simulink model "Model0"  (R2023b)
settings: Solver=VariableStepAuto  StartTime=0.0  StopTime=10.0  RelTol=1e-3
values from neighbouring files (symbols this model uses):
  A = pi*((d)^2)/4    (= 0.196349540849)    [Parameters.m]
  a = 2.2*10^-4    (= 0.00022)    [Parameters.m]
  Af = 45    [Parameters.m]
  As = 30    [Parameters.m]
  c = c_*A/L_SMA    (= 0.00981747704247)    [Parameters.m]
  c_ = 10    [Parameters.m]
  Ca = 10.3    [Parameters.m]
  Cm = 7    [Parameters.m]
  Cp = 322    [Parameters.m]
  d = 0.5    [Parameters.m]
  e_l = 0.05    [Parameters.m]
  Ea = 75000    [Parameters.m]
  Em = 28000    [Parameters.m]
  gm = I_max/V_max    (= 0.945945945946)    [Parameters.m]
  h = 36200    [Parameters.m]
  Ip = a*T0/Rp    (= 0.00210434782609)    [Parameters.m]
  k = k_*Ap/t    (= 4.26315789474)    [Parameters.m]
  L_SMA = 200    [Parameters.m]
  m = (V*10^-9)/raw    (= 6.08835785579e-12)    [Parameters.m]
  n = 3    [Parameters.m]
  R = 7.8    [Parameters.m]
  R1 = 1000    [Parameters.m]
  R2 = 1000    [Parameters.m]
  R_ = 0.000820    (= 0.00082)    [Parameters.m]
  R_load = Gv/gm    (= 2.11428571429)    [Parameters.m]
  Rp = 2.3    [Parameters.m]
  T0 = 22    [Parameters.m]
undefined symbols (not defined in the file or in its folder): K, R_int, T
libraries: fl_lib x4, ee_lib x2, nesl_utility x2
settings Model: Creator=DELL  LastModifiedBy=DELL

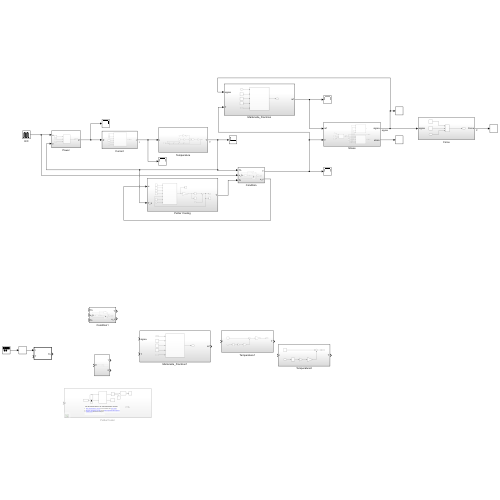
[thumbnail: Simulink's stored preview of the top-level diagram]
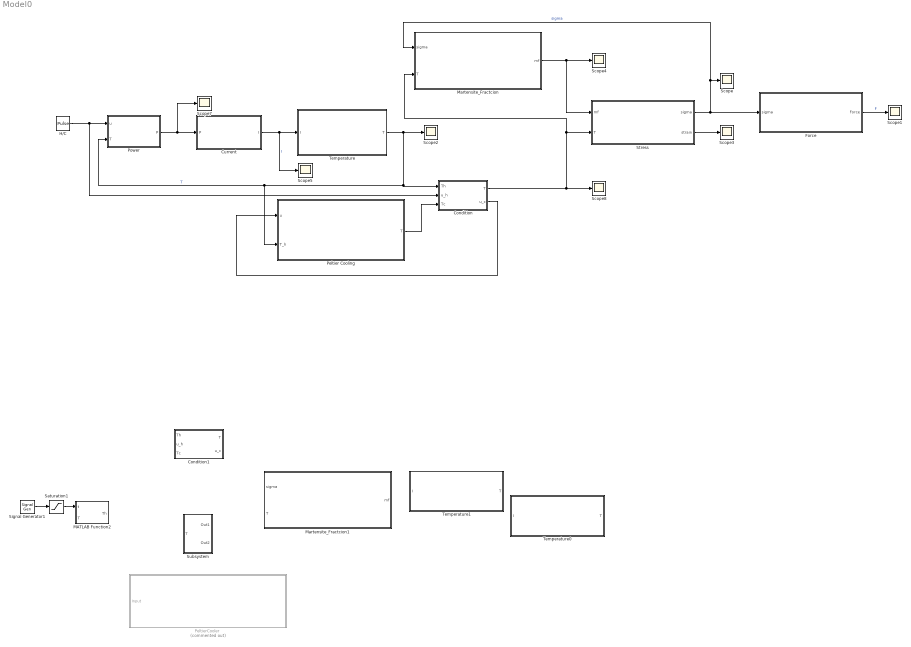
== system Model0 ==
  Condition : Subsystem
  Condition1 : Subsystem
  Current : Subsystem
  Force : Subsystem
  H/C : DiscretePulseGenerator  PulseType=Time based  Period=10  PulseWidth=50
  MATLAB Function2 : MATLAB Function  TreatAsAtomicUnit=on
  Martensite_Fractcion : Subsystem
  Martensite_Fractcion1 : Subsystem
  Peltier Cooling : Subsystem
  PeltierCooler : Subsystem  Commented=on
  Power : Subsystem
  Saturation1 : Saturate  UpperLimit=0.0578  LowerLimit=0
  Scope{,1..5,7..8} (8 alike) : Scope
  Signal Generator1 : SignalGenerator  WaveForm=square  Amplitude=-0.0578  Frequency=0.095
  Stress : Subsystem
  Subsystem : Subsystem
  Temperature : Subsystem
  Temperature0 : Subsystem
  Temperature1 : Subsystem
  wires:
  Martensite_Fractcion/1(mf) -> Scope4/1, Stress/1(mf)
  Stress/1(sigma) -> Martensite_Fractcion/1(sigma), Scope/1, Force/1(sigma)  "sigma"
  Force/1(Force) -> Scope1/1  "F"
  Temperature/1(T) -> Scope2/1, Peltier Cooling/2(T_h), Power/2(T), Condition/1(Th)  "T"
  Current/1(I) -> Temperature/1(I), Scope5/1  "I"
  Stress/2(strain) -> Scope3/1
  Signal Generator1/1 -> Saturation1/1
  Saturation1/1 -> MATLAB Function2/1(t)
  Condition/1(T) -> Martensite_Fractcion/2(T), Stress/2(T), Scope8/1
  Peltier Cooling/1(T) -> Condition/3(Tc)
  Condition/2(u_c) -> Peltier Cooling/1(u)
  Power/1(P) -> Scope7/1, Current/1(P)
  H/C/1 -> Condition/2(u_h), Power/1(u)

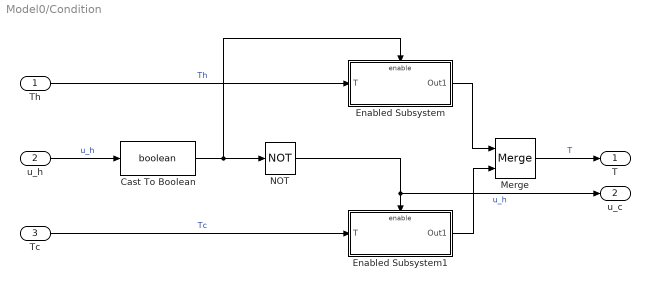
== system Model0/Condition ==
  Th : Inport
  u_h : Inport  Port=2
  Tc : Inport  Port=3
  Cast To Boolean : DataTypeConversion  OutDataTypeStr=boolean  SaturateOnIntegerOverflow=off  RndMeth=Floor
  Enabled Subsystem : Subsystem  TreatAsAtomicUnit=on
  Enabled Subsystem1 : Subsystem  TreatAsAtomicUnit=on
  Merge : Merge
  NOT : Logic  Operator=NOT  IconShape=distinctive  AllPortsSameDT=off  OutDataTypeStr=boolean
  T : Outport
  u_c : Outport  Port=2
  wires:
  Merge/1 -> T/1  "T"
  Enabled Subsystem/1(Out1) -> Merge/1
  Cast To Boolean/1 -> NOT/1, Enabled Subsystem/Enable
  NOT/1 -> u_c/1, Enabled Subsystem1/Enable  "u_h"
  Tc/1 -> Enabled Subsystem1/1(T)  "Tc"
  Th/1 -> Enabled Subsystem/1(T)  "Th"
  Enabled Subsystem1/1(Out1) -> Merge/2
  u_h/1 -> Cast To Boolean/1  "u_h"

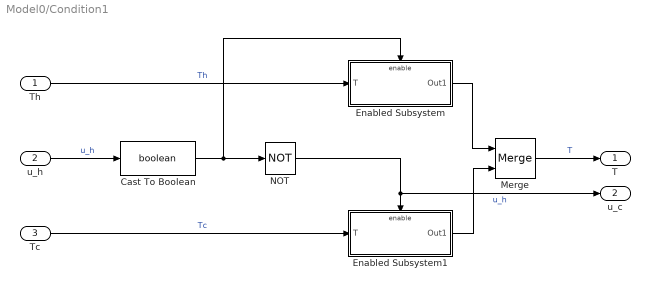
== system Model0/Condition1 ==
  Th : Inport
  u_h : Inport  Port=2
  Tc : Inport  Port=3
  Cast To Boolean : DataTypeConversion  OutDataTypeStr=boolean  SaturateOnIntegerOverflow=off  RndMeth=Floor
  Enabled Subsystem : Subsystem  TreatAsAtomicUnit=on
  Enabled Subsystem1 : Subsystem  TreatAsAtomicUnit=on
  Merge : Merge
  NOT : Logic  Operator=NOT  IconShape=distinctive  AllPortsSameDT=off  OutDataTypeStr=boolean
  T : Outport
  u_c : Outport  Port=2
  wires:
  Merge/1 -> T/1  "T"
  Enabled Subsystem/1(Out1) -> Merge/1
  Cast To Boolean/1 -> NOT/1, Enabled Subsystem/Enable
  NOT/1 -> u_c/1, Enabled Subsystem1/Enable  "u_h"
  Tc/1 -> Enabled Subsystem1/1(T)  "Tc"
  Th/1 -> Enabled Subsystem/1(T)  "Th"
  Enabled Subsystem1/1(Out1) -> Merge/2
  u_h/1 -> Cast To Boolean/1  "u_h"

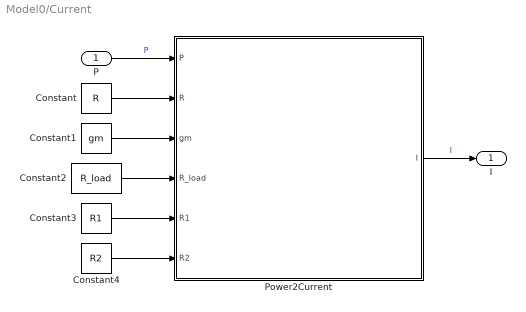
== system Model0/Current ==
  P : Inport
  Constant : Constant  Value=R
  Constant1 : Constant  Value=gm
  Constant2 : Constant  Value=R_load
  Constant3 : Constant  Value=R1
  Constant4 : Constant  Value=R2
  Power2Current : MATLAB Function  TreatAsAtomicUnit=on
  I : Outport
  wires:
  P/1 -> Power2Current/1(P)  "P"
  Power2Current/1(I) -> I/1  "I"
  Constant/1 -> Power2Current/2(R)
  Constant2/1 -> Power2Current/4(R_load)
  Constant3/1 -> Power2Current/5(R1)
  Constant4/1 -> Power2Current/6(R2)
  Constant1/1 -> Power2Current/3(gm)

== system Model0/Force ==
  sigma : Inport
  Area_SMA : Constant  Value=A
  Divide : Product  Inputs=***
  No. of Wires : Constant  Value=n
  Force : Outport
  wires:
  Area_SMA/1 -> Divide/2  "A"
  sigma/1 -> Divide/3  "sigma"
  Divide/1 -> Force/1  "F"
  No. of Wires/1 -> Divide/1  "n"

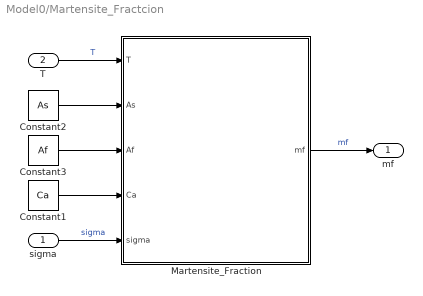
== system Model0/Martensite_Fractcion ==
  sigma : Inport
  T : Inport  Port=2
  Constant1 : Constant  Value=Ca
  Constant2 : Constant  Value=As
  Constant3 : Constant  Value=Af
  Martensite_Fraction : MATLAB Function  TreatAsAtomicUnit=on
  mf : Outport
  wires:
  sigma/1 -> Martensite_Fraction/5(sigma)  "sigma"
  Constant2/1 -> Martensite_Fraction/2(As)
  Martensite_Fraction/1(mf) -> mf/1  "mf"
  T/1 -> Martensite_Fraction/1(T)  "T"
  Constant1/1 -> Martensite_Fraction/4(Ca)
  Constant3/1 -> Martensite_Fraction/3(Af)

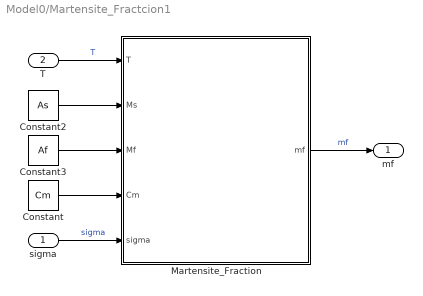
== system Model0/Martensite_Fractcion1 ==
  sigma : Inport
  T : Inport  Port=2
  Constant : Constant  Value=Cm
  Constant2 : Constant  Value=As
  Constant3 : Constant  Value=Af
  Martensite_Fraction : MATLAB Function  TreatAsAtomicUnit=on
  mf : Outport
  wires:
  sigma/1 -> Martensite_Fraction/5(sigma)  "sigma"
  Constant2/1 -> Martensite_Fraction/2(Ms)
  Martensite_Fraction/1(mf) -> mf/1  "mf"
  T/1 -> Martensite_Fraction/1(T)  "T"
  Constant/1 -> Martensite_Fraction/4(Cm)
  Constant3/1 -> Martensite_Fraction/3(Mf)

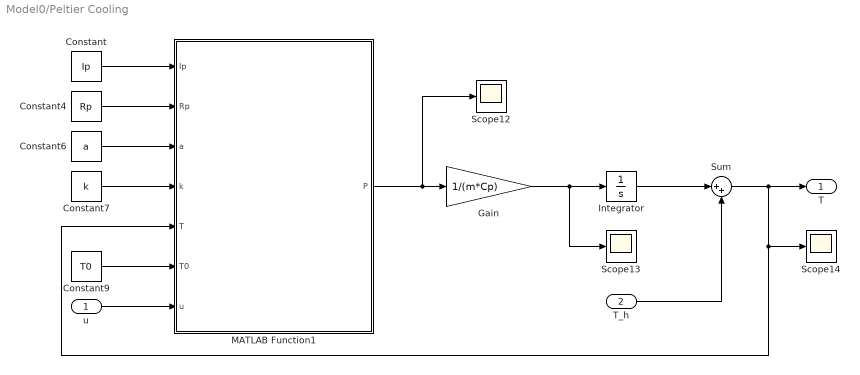
== system Model0/Peltier Cooling ==
  u : Inport
  T_h : Inport  Port=2
  Constant : Constant  Value=Ip
  Constant4 : Constant  Value=Rp
  Constant6 : Constant  Value=a
  Constant7 : Constant  Value=k
  Constant9 : Constant  Value=T0
  Gain : Gain  Gain=1/(m*Cp)
  Integrator : Integrator
  MATLAB Function1 : MATLAB Function  TreatAsAtomicUnit=on
  Scope12 : Scope
  Scope13 : Scope
  Scope14 : Scope
  Sum : Sum  Inputs=|++
  T : Outport
  wires:
  Constant4/1 -> MATLAB Function1/2(Rp)
  MATLAB Function1/1(P) -> Scope12/1, Gain/1
  Constant6/1 -> MATLAB Function1/3(a)
  T_h/1 -> Sum/2
  u/1 -> MATLAB Function1/7(u)
  Constant9/1 -> MATLAB Function1/6(T0)
  Constant/1 -> MATLAB Function1/1(Ip)
  Integrator/1 -> Sum/1
  Sum/1 -> T/1, MATLAB Function1/5(T), Scope14/1
  Gain/1 -> Scope13/1, Integrator/1
  Constant7/1 -> MATLAB Function1/4(k)

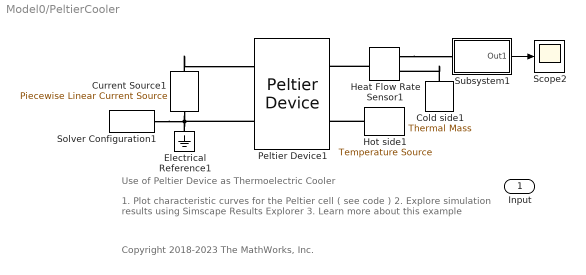
== system Model0/PeltierCooler ==
  note: Copyright 2018-2023 The MathWorks, Inc.
  note: 1. Plot characteristic curves for the Peltier cell ( see code )
      | 2. Explore simulation results using Simscape Results Explorer
      | 3. Learn more about this example
  note: Use of Peltier Device as Thermoelectric Cooler
  Input : Inport
  Cold side1 : fl_lib/Thermal/Thermal Elements/Thermal Mass  mass_type=foundation.enum.constant_variable.constant  mass=1 kg  sp_heat=447 J/kg/K  mass_min=1e-6 kg  num_ports=foundation.enum.numPorts2.one  m_specify=off  m_priority=High  m=1 kg  m_nominal_specify=off  m_nominal_unit=kg  m_nominal_value=1  T_specify=on  T_priority=High  T=T K  T_nominal_specify=off  T_nominal_unit=K  T_nominal_value=1  Q_specify=off  Q_priority=None  Q=0 W  Q_nominal_specify=off  Q_nominal_unit=W  Q_nominal_value=1
  Current Source1 : ee_lib/Additional Components/SPICE Sources/Piecewise Linear Current Source  TIMElist=[0, 10] s  CURRlist=[0.01, 5.5] A  INTERP=1  EXTRAP=1  Gmin_param=ee.enum.gminParam.yes
      settings: InternalSimscapePortConfiguration="{\"Bottom\":[],\"Left\":[{\"id\":\"p\",\"label\":\"+\",\"type\":\"foundation.electrical.electrical\"}],\"Right\":[{\"id\":\"n\",\"label\":\"-\",\"type\":\"foundation.electrical.electrical\"}],\"Top\":[]}"
  Electrical Reference1 : fl_lib/Electrical/Electrical Elements/Electrical Reference
  Heat Flow Rate Sensor1 : fl_lib/Thermal/Thermal Sensors/Heat Flow Rate Sensor
  Hot side1 : fl_lib/Thermal/Thermal Sources/Temperature Source  temperature=323.15 K
  Peltier Device1 : ee_lib/Sensors & Transducers/Peltier Device  alpha="coef  V/K"  R="R_int  Ohm"  K=K W/K
      settings: InternalSimscapePortConfiguration="{\"Bottom\":[],\"Left\":[{\"id\":\"p\",\"label\":\"+\",\"type\":\"foundation.electrical.electrical\"},{\"id\":\"n\",\"label\":\"-\",\"type\":\"foundation.electrical.electrical\"}],\"Right\":[{\"id\":\"A\",\"label\":\"A\",\"type\":\"foundation.thermal.thermal\"},{\"id\":\"B\",\"label\":\"B\",\"type\":\"foundation.thermal.thermal\"}],\"Top\":[]}"
  Scope2 : Scope
  Solver Configuration1 : nesl_utility/Solver Configuration  PhysicalDomain=network_engine_domain  SubClassName=solver  LeftPortType=input  RightPortType=generic  Tones=[]  Harmonics=[]  SimulateNoise=off  Profile=off  UseLocalSampling=off  EnableSwitchedLinearOptims=on  FrequencyDomain=off  UseCCode=off  RelTol=0.001  AbsTol=1e-06  MinStep=1e-09  ToWorkspace=off  RevertToSquareIcSolve=off  NumHomotopyIterations=100  PhasorMode=off  PhasorModeNumHarmonics=1  ConsistencySolver=NEWTON_FTOL  IndexReductionMethod=DerivativeReplacement  DoDC=off  ResidualTolerance=1e-09  ConsistencyTolSource=GLOBAL  ConsistencyAbsTol=0.001  ConsistencyRelTol=0.001  ConsistencyTolFactor=0.001  UseLocalSolver=off  LocalSolverChoice=NE_BACKWARD_EULER_ADVANCER  ResolveIndetEquations=on  FunctionEvalNumThread=1  LocalSolverSampleTime=0.001  DoFixedCost=off  MaxNonlinIter=3  MaxModeIter=2  ComputeImpulses=off  ImpulseIterations=2  LinearAlgebra=auto  LinearAlgebraNumThread=0  EquationFormulation=NE_TIME_EF  DelaysMemoryBudget=1024  AutomaticFiltering=on  FilteringTimeConstant=0.001  PartitionStorageMethod=AS_NEEDED  PartitionMemoryBudget=1024  PartitionMethod=FAST  MultibodyUseLocalSolver=off  MultibodyLocalSolverChoice=ODE1  MultibodyLocalSolverSampleTime=0.001
  Subsystem1 : Subsystem
      mask Display: disp('Heat flow')
  wires:
  Subsystem1/1(Out1) -> Scope2/1
  connections:
  Heat Flow Rate Sensor1/LConn1 -- Peltier Device1/RConn1
  Current Source1/LConn1 -- Solver Configuration1/RConn1 -- Electrical Reference1/LConn1 -- Peltier Device1/LConn2
  Heat Flow Rate Sensor1/RConn1 -- Subsystem1/LConn1
  Cold side1/LConn1 -- Heat Flow Rate Sensor1/RConn2
  Hot side1/LConn1 -- Peltier Device1/RConn2
  Current Source1/RConn1 -- Peltier Device1/LConn1

== system Model0/Power ==
  u : Inport
  T : Inport  Port=2
  MATLAB Function1 : MATLAB Function  TreatAsAtomicUnit=on
  Step : Step  After=0.0578  SampleTime=0
  P : Outport
  wires:
  T/1 -> MATLAB Function1/3(T)  "T"
  MATLAB Function1/1(P) -> P/1  "P"
  Step/1 -> MATLAB Function1/1(p)  "P"
  u/1 -> MATLAB Function1/2(u)  "u"

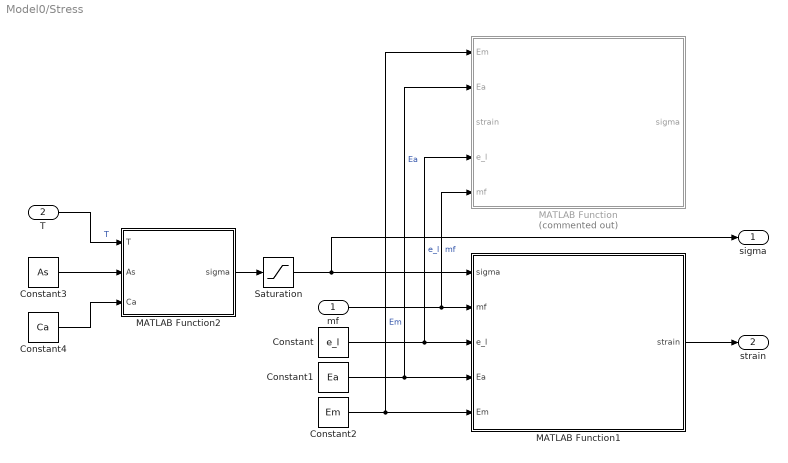
== system Model0/Stress ==
  mf : Inport
  T : Inport  Port=2
  Constant : Constant  Value=e_l
  Constant1 : Constant  Value=Ea
  Constant2 : Constant  Value=Em
  Constant3 : Constant  Value=As
  Constant4 : Constant  Value=Ca
  MATLAB Function : MATLAB Function  Commented=on  TreatAsAtomicUnit=on
  MATLAB Function1 : MATLAB Function  TreatAsAtomicUnit=on
  MATLAB Function2 : MATLAB Function  TreatAsAtomicUnit=on
  Saturation : Saturate  UpperLimit=170  LowerLimit=0
  sigma : Outport
  strain : Outport  Port=2
  wires:
  Constant2/1 -> MATLAB Function/1(Em), MATLAB Function1/5(Em)  "Em"
  Constant1/1 -> MATLAB Function/2(Ea), MATLAB Function1/4(Ea)  "Ea"
  Constant/1 -> MATLAB Function/4(e_l), MATLAB Function1/3(e_l)  "e_l"
  mf/1 -> MATLAB Function/5(mf), MATLAB Function1/2(mf)  "mf"
  MATLAB Function2/1(sigma) -> Saturation/1
  T/1 -> MATLAB Function2/1(T)  "T"
  Constant3/1 -> MATLAB Function2/2(As)
  Constant4/1 -> MATLAB Function2/3(Ca)
  MATLAB Function1/1(strain) -> strain/1
  Saturation/1 -> sigma/1, MATLAB Function1/1(sigma)

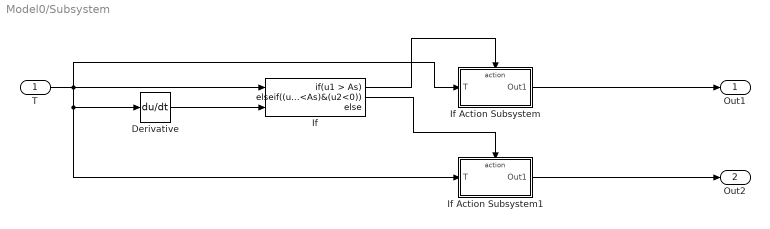
== system Model0/Subsystem ==
  T : Inport
  Derivative : Derivative
  If : If  NumInputs=2  IfExpression=u1 > As  ElseIfExpressions=(u1<As)&(u2<0)
  If Action Subsystem : Subsystem  TreatAsAtomicUnit=on
  If Action Subsystem1 : Subsystem  TreatAsAtomicUnit=on
  Out1 : Outport
  Out2 : Outport  Port=2
  wires:
  If Action Subsystem/1(Out1) -> Out1/1
  Derivative/1 -> If/2
  T/1 -> If Action Subsystem/1(T), If Action Subsystem1/1(T), Derivative/1, If/1
  If Action Subsystem1/1(Out1) -> Out2/1
  If/2 -> If Action Subsystem1/Action
  If/1 -> If Action Subsystem/Action

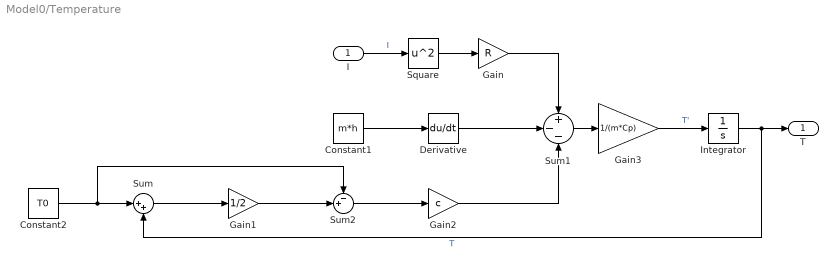
== system Model0/Temperature ==
  I : Inport
  Constant1 : Constant  Value=m*h
  Constant2 : Constant  Value=T0
  Derivative : Derivative
  Gain : Gain  Gain=R
  Gain1 : Gain  Gain=1/2
  Gain2 : Gain  Gain=c
  Gain3 : Gain  Gain=1/(m*Cp)
  Integrator : Integrator
  Square : Math  Operator=square
  Sum : Sum  Inputs=|++
  Sum1 : Sum  Inputs=+--
  Sum2 : Sum  Inputs=-+|
  T : Outport
  wires:
  Constant1/1 -> Derivative/1
  Square/1 -> Gain/1
  Sum1/1 -> Gain3/1
  I/1 -> Square/1  "I"
  Gain/1 -> Sum1/1
  Integrator/1 -> Sum/2, T/1  "T"
  Gain3/1 -> Integrator/1  "T'"
  Derivative/1 -> Sum1/2
  Constant2/1 -> Sum2/1, Sum/1
  Sum/1 -> Gain1/1
  Gain1/1 -> Sum2/2
  Sum2/1 -> Gain2/1
  Gain2/1 -> Sum1/3

== system Model0/Temperature0 ==
  I : Inport
  Constant1 : Constant  Value=T0
  Gain : Gain  Gain=R_
  Gain1 : Gain  Gain=1/((pi^2)*((d/1000)^3)*(c_*1000/L_SMA))
  Square : Math  Operator=square
  Sum : Sum  Inputs=|++
  T : Outport
  wires:
  Square/1 -> Gain/1
  Gain1/1 -> Sum/2
  I/1 -> Square/1  "I"
  Sum/1 -> T/1
  Gain/1 -> Gain1/1
  Constant1/1 -> Sum/1

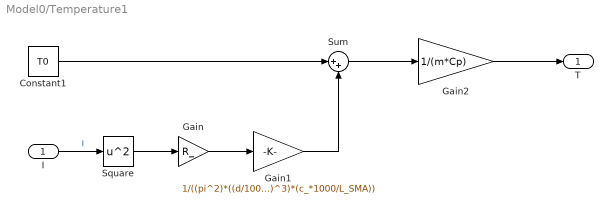
== system Model0/Temperature1 ==
  I : Inport
  Constant1 : Constant  Value=T0
  Gain : Gain  Gain=R_
  Gain1 : Gain  Gain=1/((pi^2)*((d/1000)^3)*(c_*1000/L_SMA))
  Gain2 : Gain  Gain=1/(m*Cp)
  Square : Math  Operator=square
  Sum : Sum  Inputs=|++
  T : Outport
  wires:
  Square/1 -> Gain/1
  Gain1/1 -> Sum/2
  I/1 -> Square/1  "I"
  Sum/1 -> Gain2/1
  Gain/1 -> Gain1/1
  Constant1/1 -> Sum/1
  Gain2/1 -> T/1

== system Model0/Condition/Enabled Subsystem ==
  T : Inport
  Enable : EnablePort
  Out1 : Outport
  wires:
  T/1 -> Out1/1

== system Model0/Condition/Enabled Subsystem1 ==
  T : Inport
  Enable : EnablePort
  Out1 : Outport
  wires:
  T/1 -> Out1/1

== system Model0/Condition1/Enabled Subsystem ==
  T : Inport
  Enable : EnablePort
  Out1 : Outport
  wires:
  T/1 -> Out1/1

== system Model0/Condition1/Enabled Subsystem1 ==
  T : Inport
  Enable : EnablePort
  Out1 : Outport
  wires:
  T/1 -> Out1/1

== system Model0/PeltierCooler/Subsystem1 ==
  Gain : Gain  Gain=-1
  PS-Simulink Converter : nesl_utility/PS-Simulink Converter  PhysicalDomain=network_engine_domain  SubClassName=ps_output  LeftPortType=input  RightPortType=output  PseudoPeriodic=off  Frequencies=[]  VectorFormat=1-D array  Unit=J/s  AffineConversion=off
  Conn1 : PMIOPort  Side=Left
  Out1 : Outport  VectorParamsAs1DForOutWhenUnconnected=off
  wires:
  Gain/1 -> Out1/1
  PS-Simulink Converter/1 -> Gain/1
  connections:
  Conn1/RConn1 -- PS-Simulink Converter/LConn1

== system Model0/Subsystem/If Action Subsystem ==
  T : Inport
  Action Port : ActionPort  ActionPortLabel=if(u1 > As)
  Out1 : Outport
  wires:
  T/1 -> Out1/1

== system Model0/Subsystem/If Action Subsystem1 ==
  T : Inport
  Action Port : ActionPort  ActionPortLabel=elseif((u1<As)&(u2<0))
  Out1 : Outport
  wires:
  T/1 -> Out1/1

== matlab function Model0/MATLAB Function2 ==
  data: t input; T input; Th output
function Th = fcn(t, T)

if (t~=0)
    Th = T;
else
    Th = 45;
end

== matlab function Model0/Martensite_Fractcion/Martensite_Fraction ==
  data: T input; As input; Af input; Ca input; sigma input; mf output
function mf = fcn(T, As, Af, Ca, sigma)

%mf = 1- exp(Ca*(T-As)+Cm*sigma);
%mf = 1- exp(log(0.01)*(As-T)/(As-Af)+sigma*log(0.01)/(Ca*(As-Af)));
if T>As
    mf = 1-(1/2)*(cos(pi*(T-As)/(Af-As)-pi*sigma/(Ca*(Af-As)))+1);
else
    mf = 1;
end

== matlab function Model0/Stress/MATLAB Function ==
  data: Em input; sigma output; Ea input; strain input; e_l input; mf input
function sigma = fcn(Em, Ea, strain, e_l, mf)

E = Em*mf + Ea*(1-mf);

sigma = E*strain - e_l*mf;

== matlab function Model0/Current/Power2Current ==
  data: P input; I output; R input; gm input; R_load input; R1 input; R2 input
function I = fcn(P,R, gm, R_load, R1, R2)

I_req = sqrt(P/R);
V_in = I_req/gm;
Gv = (1+R1/R2);
V_out = V_in*Gv;

I = V_out/R_load;

== matlab function Model0/Stress/MATLAB Function1 ==
  data: sigma input; strain output; mf input; e_l input; Ea input; Em input
function strain = fcn(sigma, mf, e_l, Ea, Em)

E = Em*mf + Ea*(1-mf);

strain = (sigma/E) + e_l*mf;

== matlab function Model0/Stress/MATLAB Function2 ==
  data: T input; sigma output; As input; Ca input
function sigma = fcn(T, As, Ca)

sigma = Ca * (T-As);

== matlab function Model0/Martensite_Fractcion1/Martensite_Fraction ==
  data: T input; Ms input; Mf input; Cm input; sigma input; mf output
function mf = fcn(T, Ms, Mf, Cm, sigma)

if T<Ms
    mf = 1 - (1/2)*cos(pi*(T-Ms)/(Mf-Ms)-pi*sigma/(Cm*(Mf-Ms))) + (1/2);
else
    mf = 0;
end

== matlab function Model0/Peltier Cooling/MATLAB Function1 ==
  data: Ip input; P output; Rp input; a input; k input; T input; T0 input; u input
function P = fcn(Ip, Rp, a, k, T, T0, u)

Tc = T0;

if (T>T0)&&(u==0)
    I = Ip;
else
    I = 0;
end

P = (1/12)*(I^2)*Rp - a*I*T;% - k*(Th-Tc);

== matlab function Model0/Power/MATLAB Function1 ==
  data: p input; u input; T input; P output
function P = fcn(p, u, T)

if (T<45)&&(u==1)
    P = p;
else
    P = 0;
end
